simulink model "SimpleDigitalDesignSLX"  (R2021a)
settings: Solver=ode1  StartTime=0.0  StopTime=10.0  FixedStep=1e-4  RelTol=1e-3
InitFcn:
  | SimpleDigitalDesign
StartFcn:
  | SimpleDigitalDesign
values from neighbouring files (symbols this model uses):
  T = 0.04    [SimpleDigitalDesign.m]
  To = 0.2    [SimpleDigitalDesign.m]
undefined symbols (not defined in the file or in its folder): Acd, Bcd, Ccd, Dcd
settings Model: Creator=aghersin  LastModifiedBy=aghersin
settings SolverCC: AlgebraicLoopSolver=TrustRegion
settings DataIOCC: ReturnWorkspaceOutputs=off
settings DebuggingCC: SFMachineParentedDataDiag=warning  ArithmeticOperatorsInVariantConditions=warning
settings SFSimCC: SimUseLocalCustomCode=off  CustomCodeUndefinedFunction=UseInterfaceOnly
settings RTWCC: RTWUseLocalCustomCode=off

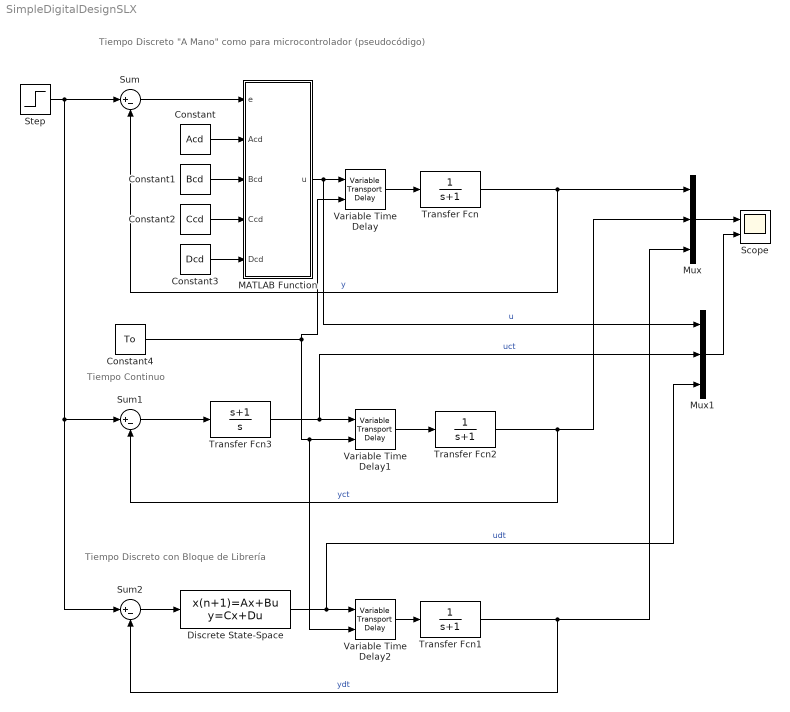
== system SimpleDigitalDesignSLX ==
  note: Tiempo Discreto "A Mano" como para microcontrolador (pseudocódigo)
  note: Tiempo Discreto con Bloque de Librería
  note: Tiempo Continuo
  Constant : Constant  Value=Acd
  Constant1 : Constant  Value=Bcd
  Constant2 : Constant  Value=Ccd
  Constant3 : Constant  Value=Dcd
  Constant4 : Constant  Value=To
  Discrete State-Space : DiscreteStateSpace  A=Acd  B=Bcd  C=Ccd  D=Dcd  SampleTime=T
  MATLAB Function : MATLAB Function  TreatAsAtomicUnit=on  SystemSampleTime=T
  Mux : Mux  Inputs=3
  Mux1 : Mux  Inputs=3
  Scope : Scope  NumInputPorts=2
  Step : Step  SampleTime=0
  Sum : Sum  Inputs=|+-
  Sum1 : Sum  Inputs=|+-
  Sum2 : Sum  Inputs=|+-
  Transfer Fcn : TransferFcn  Denominator=[1 1]
  Transfer Fcn1 : TransferFcn  Denominator=[1 1]
  Transfer Fcn2 : TransferFcn  Denominator=[1 1]
  Transfer Fcn3 : TransferFcn  Numerator=[1 1]  Denominator=[1 0]
  Variable Time Delay : VariableTransportDelay  MaximumDelay=10
  Variable Time Delay1 : VariableTransportDelay  MaximumDelay=10
  Variable Time Delay2 : VariableTransportDelay  MaximumDelay=10
  wires:
  Variable Time Delay/1 -> Transfer Fcn/1
  Constant/1 -> MATLAB Function/2(Acd)
  Constant1/1 -> MATLAB Function/3(Bcd)
  Constant2/1 -> MATLAB Function/4(Ccd)
  Constant3/1 -> MATLAB Function/5(Dcd)
  MATLAB Function/1(u) -> Variable Time Delay/1, Mux1/1  "u"
  Sum/1 -> MATLAB Function/1(e)
  Transfer Fcn/1 -> Mux/1, Sum/2  "y"
  Transfer Fcn2/1 -> Mux/2, Sum1/2  "yct"
  Transfer Fcn3/1 -> Variable Time Delay1/1, Mux1/2  "uct"
  Variable Time Delay1/1 -> Transfer Fcn2/1
  Sum1/1 -> Transfer Fcn3/1
  Variable Time Delay2/1 -> Transfer Fcn1/1
  Step/1 -> Sum2/1, Sum1/1, Sum/1
  Discrete State-Space/1 -> Mux1/3, Variable Time Delay2/1  "udt"
  Sum2/1 -> Discrete State-Space/1
  Transfer Fcn1/1 -> Sum2/2, Mux/3  "ydt"
  Mux/1 -> Scope/1
  Mux1/1 -> Scope/2
  Constant4/1 -> Variable Time Delay/2, Variable Time Delay2/2, Variable Time Delay1/2

== matlab function SimpleDigitalDesignSLX/MATLAB Function ==
  data: e input; u output; Acd input; Bcd input; Ccd input; Dcd input
function u = controller(e,Acd,Bcd,Ccd,Dcd)

persistent xcd

if isempty(xcd)
    xcd = 0;
end

% Si implementáramos en microcontrolador:
% muestreamos "e" cada "T" segundos con el conversor A/D.
% actualizamos "u" cada "T" segundos con el conversor D/A.

xcd1=Acd*xcd+Bcd*e;
u=Ccd*xcd+Dcd*e;

xcd=xcd1;
end
